simulink model "ESP_TCP_scoring"  (R2023a)
settings: Solver=FixedStepAuto  StartTime=0.0  StopTime=90  FixedStep=1  RelTol=1e-3
libraries: simulink x61, instrumentlib x2, dspsigattribs x1, dspstat3 x1, slrealtimeiplib x1
settings Model: SimulationMode=accelerator  PacingRate=6  Creator=Acer  LastModifiedBy=Acer

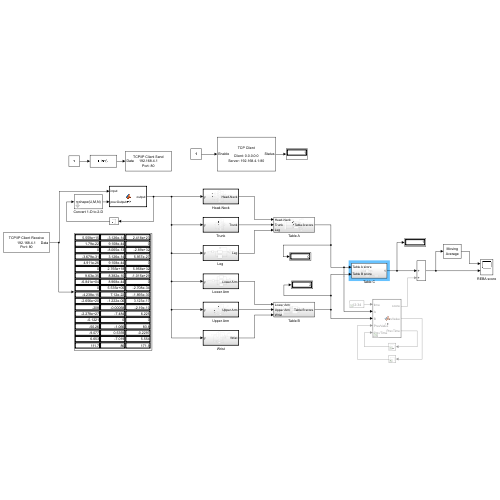
[thumbnail: Simulink's stored preview of the top-level diagram]
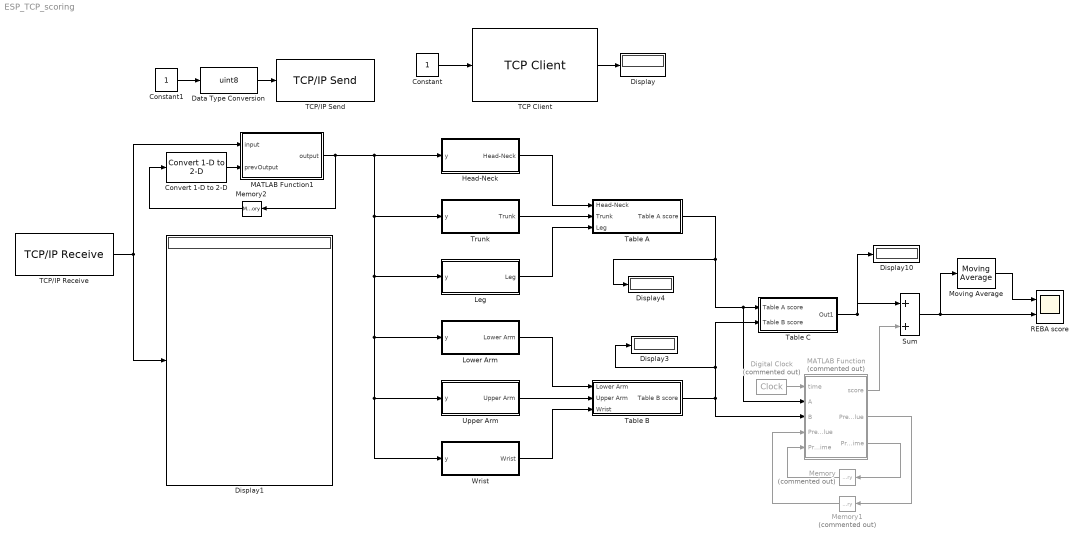
== system ESP_TCP_scoring ==
  Constant : Constant
  Constant1 : Constant
  Convert 1-D to 2-D : dspsigattribs/Convert 1-D to 2-D  M=1  N=54  frameBasedOut=off
      settings: LibrarySourceBlock=dsphdlsupportsigmgmt/Convert 1-D to 2-D
  Data Type Conversion : DataTypeConversion  OutDataTypeStr=uint8  SaturateOnIntegerOverflow=off  RndMeth=Floor
  Digital Clock : DigitalClock  Commented=on
  Display{,1,3..4,10} (5 alike) : Display
  Head-Neck : Subsystem  TreatAsAtomicUnit=on
  "Leg " : Subsystem  TreatAsAtomicUnit=on
  Lower Arm : Subsystem  TreatAsAtomicUnit=on
  MATLAB Function : MATLAB Function  Commented=on  TreatAsAtomicUnit=on
  MATLAB Function1 : MATLAB Function  TreatAsAtomicUnit=on
  Memory : Memory  Commented=on
  Memory1 : Memory  Commented=on
  Memory2 : Memory  InitialCondition=zeros(1,54)
  Moving Average : dspstat3/Moving Average  Method=Sliding window  ForgettingFactorPort=off  SpecifyWindowLength=on  WindowLength=4  OverlapLength=3  AllowArbitraryInputLength=off  ForgettingFactor=0.9  SimulateUsing=Code generation
  REBA score : Scope  NumInputPorts=2
  Sum : Sum  Inputs=|++
  TCP Client : slrealtimeiplib/TCP Client  Priority=-1  useHostTargetConn=off  remoteAddress=192.168.4.1  remotePort=80
  TCP/IP Receive : instrumentlib/TCP//IP Receive  Host=192.168.4.1  Port=80  DataSize=[ 1, 54]  DataType=double  ASCIIFormatting=%f  Terminator=LF  CustomTerminator=10  ByteOrder=little-endian  EnableBlockingMode=on  Timeout=20  SampleTime=1  SimulateUsing=Interpreted execution
  TCP/IP Send : instrumentlib/TCP//IP Send  Host=192.168.4.1  Port=80  ByteOrder=big-endian  EnableBlockingMode=on  Timeout=20  TransferDelay=on  SimulateUsing=Interpreted execution
  Table A : Subsystem
  Table B : Subsystem
  Table C : Subsystem
  Trunk : Subsystem  TreatAsAtomicUnit=on
  Upper Arm : Subsystem  TreatAsAtomicUnit=on
  Wrist : Subsystem  TreatAsAtomicUnit=on
  wires:
  Constant1/1 -> Data Type Conversion/1
  Constant/1 -> TCP Client/1
  Data Type Conversion/1 -> TCP/IP Send/1
  TCP Client/1 -> Display/1
  TCP/IP Receive/1 -> Display1/1, MATLAB Function1/1(input)
  Head-Neck/1(Head-Neck) -> Table A/1(Head-Neck)
  Trunk/1(Trunk) -> Table A/2(Trunk)
  "Leg "/1(Leg) -> Table A/3(Leg)
  Lower Arm/1(Lower Arm) -> Table B/1(Lower Arm)
  Upper Arm/1(Upper Arm) -> Table B/2(Upper Arm)
  Wrist/1(Wrist) -> Table B/3(Wrist)
  Table A/1(Table A score) -> Display4/1, MATLAB Function/2(A), Table C/1(Table A score)
  Table B/1(Table B score) -> MATLAB Function/3(B), Display3/1, Table C/2(Table B score)
  MATLAB Function/1(score) -> Sum/2
  Digital Clock/1 -> MATLAB Function/1(time)
  MATLAB Function/3(PrevTime) -> Memory/1
  Memory/1 -> MATLAB Function/5("PrevTime ")
  Memory1/1 -> MATLAB Function/4("PrevValue ")
  MATLAB Function/2(PrevValue) -> Memory1/1
  MATLAB Function1/1(output) -> Memory2/1, "Leg "/1(y), Lower Arm/1(y), Wrist/1(y), Upper Arm/1(y), Trunk/1(y), Head-Neck/1(y)
  Convert 1-D to 2-D/1 -> MATLAB Function1/2(prevOutput)
  Memory2/1 -> Convert 1-D to 2-D/1
  Table C/1(Out1) -> Sum/1, Display10/1
  Moving Average/1 -> REBA score/1
  Sum/1 -> Moving Average/1, REBA score/2

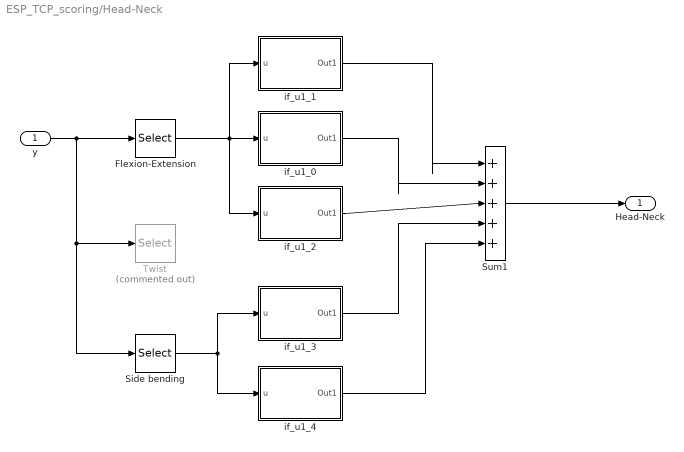
== system ESP_TCP_scoring/Head-Neck ==
  y : Inport
  Flexion-Extension : Selector  NumberOfDimensions=2  InputPortWidth=3  IndexOptions=Index vector (dialog),Index vector (dialog)  Indices=1,7  OutputSizes=1,1
  Side bending : Selector  NumberOfDimensions=2  InputPortWidth=3  IndexOptions=Index vector (dialog),Index vector (dialog)  Indices=1,1  OutputSizes=1,1
  Sum1 : Sum  Inputs=|+++++
  Twist : Selector  Commented=on  NumberOfDimensions=2  InputPortWidth=3  IndexOptions=Index vector (dialog),Index vector (dialog)  Indices=1,7  OutputSizes=1,1
  if_u1_0 : Subsystem  mask{a=69, b=1, c=2}
      mask prompts: a "u1 less then or equal to"; b "u1 greater then or equal to"; c "Constant"
      mask Display: text(5, 10, 'Gain');
  if_u1_1 : Subsystem  mask{a=80, b=70, c=1}
      mask prompts: a "u1 less then or equal to"; b "u1 greater then or equal to"; c "Constant"
      mask Display: text(5, 10, 'Gain');
  if_u1_2 : Subsystem  mask{a=180, b=100, c=2}
      mask prompts: a "u1 less then or equal to"; b "u1 greater then or equal to"; c "Constant"
      mask Display: text(5, 10, 'Gain');
  if_u1_3 : Subsystem  mask{a=-4.15, b=-9.81, c=1}
      mask prompts: a "u1 less then or equal to"; b "u1 greater then or equal to"; c "Constant"
      mask Display: text(5, 10, 'Gain');
  if_u1_4 : Subsystem  mask{a=9.81, b=4.15, c=1}
      mask prompts: a "u1 less then or equal to"; b "u1 greater then or equal to"; c "Constant"
      mask Display: text(5, 10, 'Gain');
  Head-Neck : Outport
  wires:
  y/1 -> Twist/1, Side bending/1, Flexion-Extension/1
  Flexion-Extension/1 -> if_u1_2/1(u), if_u1_0/1(u), if_u1_1/1(u)
  Side bending/1 -> if_u1_4/1(u), if_u1_3/1(u)
  if_u1_1/1(Out1) -> Sum1/1
  if_u1_0/1(Out1) -> Sum1/2
  if_u1_2/1(Out1) -> Sum1/3
  if_u1_3/1(Out1) -> Sum1/4
  if_u1_4/1(Out1) -> Sum1/5
  Sum1/1 -> Head-Neck/1

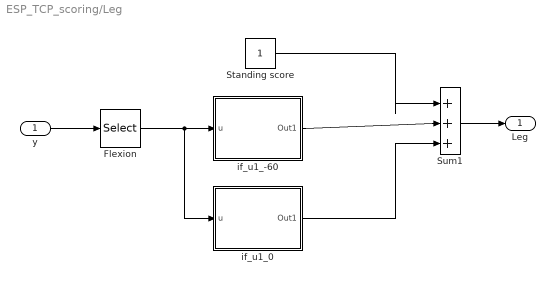
== system ESP_TCP_scoring/Leg  ==
  y : Inport
  Flexion : Selector  NumberOfDimensions=2  InputPortWidth=3  IndexOptions=Index vector (dialog),Index vector (dialog)  Indices=1,25  OutputSizes=1,1
  Standing score : Constant
  Sum1 : Sum  Inputs=|+++
  if_u1_-60 : Subsystem  mask{a=-60, b=-85, c=1}
      mask prompts: a "u1 less then or equal to"; b "u1 greater then or equal to"; c "Constant"
      mask Display: text(5, 10, 'Gain');
  if_u1_0 : Subsystem  mask{a=0, b=-59, c=2}
      mask prompts: a "u1 less then or equal to"; b "u1 greater then or equal to"; c "Constant"
      mask Display: text(5, 10, 'Gain');
  Leg : Outport
  wires:
  Standing score/1 -> Sum1/1
  y/1 -> Flexion/1
  Flexion/1 -> if_u1_0/1(u), if_u1_-60/1(u)
  if_u1_-60/1(Out1) -> Sum1/2
  if_u1_0/1(Out1) -> Sum1/3
  Sum1/1 -> Leg/1

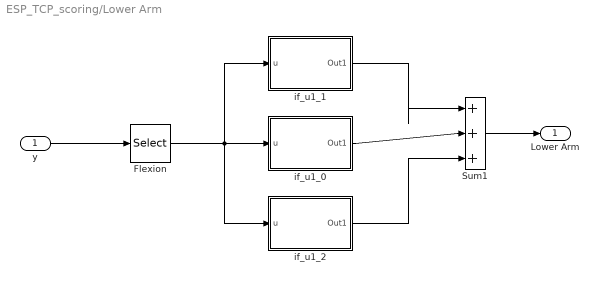
== system ESP_TCP_scoring/Lower Arm ==
  y : Inport
  Flexion : Selector  NumberOfDimensions=2  InputPortWidth=3  IndexOptions=Index vector (dialog),Index vector (dialog)  Indices=1,29  OutputSizes=1,1
  Sum1 : Sum  Inputs=|+++
  if_u1_0 : Subsystem  mask{a=9.81, b=1.71, c=2}
      mask prompts: a "u1 less then or equal to"; b "u1 greater then or equal to"; c "Constant"
      mask Display: text(5, 10, 'Gain');
  if_u1_1 : Subsystem  mask{a=1.70, b=-4.91, c=1}
      mask prompts: a "u1 less then or equal to"; b "u1 greater then or equal to"; c "Constant"
      mask Display: text(5, 10, 'Gain');
  if_u1_2 : Subsystem  mask{a=-4.91, b=-9.81, c=2}
      mask prompts: a "u1 less then or equal to"; b "u1 greater then or equal to"; c "Constant"
      mask Display: text(5, 10, 'Gain');
  Lower Arm : Outport
  wires:
  y/1 -> Flexion/1
  Flexion/1 -> if_u1_1/1(u), if_u1_0/1(u), if_u1_2/1(u)
  Sum1/1 -> Lower Arm/1
  if_u1_2/1(Out1) -> Sum1/3
  if_u1_0/1(Out1) -> Sum1/2
  if_u1_1/1(Out1) -> Sum1/1

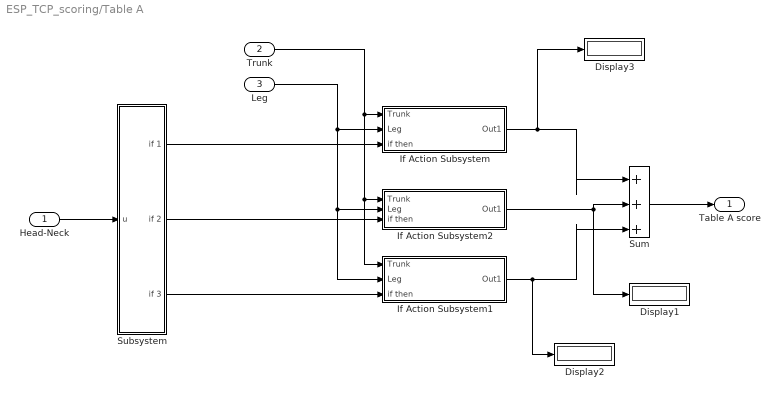
== system ESP_TCP_scoring/Table A ==
  Head-Neck : Inport
  Trunk : Inport  Port=2
  Leg : Inport  Port=3
  Display1 : Display
  Display2 : Display
  Display3 : Display
  If Action Subsystem : Subsystem  TreatAsAtomicUnit=on
  If Action Subsystem1 : Subsystem  TreatAsAtomicUnit=on
  If Action Subsystem2 : Subsystem  TreatAsAtomicUnit=on
  Subsystem : Subsystem
  Sum : Sum  Inputs=|+++
  Table A score : Outport
  wires:
  Trunk/1 -> If Action Subsystem1/1(Trunk), If Action Subsystem2/1(Trunk), If Action Subsystem/1(Trunk)
  Leg/1 -> If Action Subsystem1/2(Leg), If Action Subsystem2/2(Leg), If Action Subsystem/2(Leg)
  Sum/1 -> Table A score/1
  If Action Subsystem/1(Out1) -> Display3/1, Sum/1
  If Action Subsystem1/1(Out1) -> Display2/1, Sum/3
  Head-Neck/1 -> Subsystem/1(u)
  Subsystem/1(if 1) -> If Action Subsystem/3(if then)
  Subsystem/2(if 2) -> If Action Subsystem2/3(if then)
  Subsystem/3(if 3) -> If Action Subsystem1/3(if then)
  If Action Subsystem2/1(Out1) -> Display1/1, Sum/2

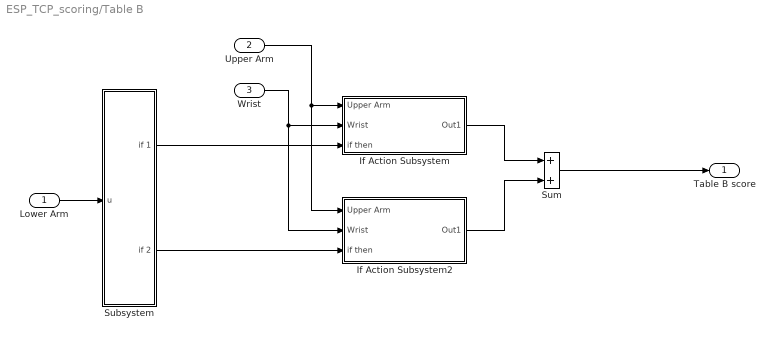
== system ESP_TCP_scoring/Table B ==
  Lower Arm : Inport
  Upper Arm : Inport  Port=2
  Wrist : Inport  Port=3
  If Action Subsystem : Subsystem  TreatAsAtomicUnit=on
  If Action Subsystem2 : Subsystem  TreatAsAtomicUnit=on
  Subsystem : Subsystem
  Sum : Sum
  Table B score : Outport
  wires:
  Upper Arm/1 -> If Action Subsystem2/1(Upper Arm), If Action Subsystem/1(Upper Arm)
  Wrist/1 -> If Action Subsystem2/2(Wrist), If Action Subsystem/2(Wrist)
  If Action Subsystem/1(Out1) -> Sum/1
  If Action Subsystem2/1(Out1) -> Sum/2
  Lower Arm/1 -> Subsystem/1(u)
  Subsystem/1(if 1) -> If Action Subsystem/3(if then)
  Subsystem/2(if 2) -> If Action Subsystem2/3(if then)
  Sum/1 -> Table B score/1

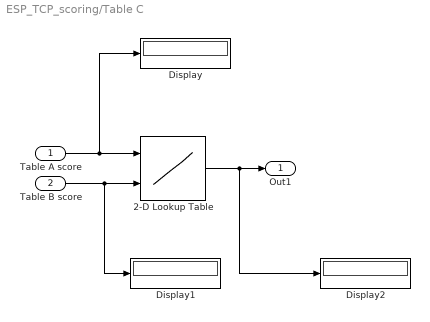
== system ESP_TCP_scoring/Table C ==
  Table A score : Inport
  Table B score : Inport  Port=2
  2-D Lookup Table : Lookup_n-D  BreakpointsForDimension1=[0:12]  BreakpointsForDimension2=[0:12]  Table=[1 1 1 1 1 1 1 1 1 1 1 1 1; 1 1 1 1 2 3 3 4 5 6 7 7 7; 1 1 2 2 3 4 4 5 6 6 7 7 8; 1 2 3 3 3 4 5 6 7 7 8 8 8; 1 3 4 4 4 5 6 7 8 8 9 9 9; 1 4 4 4 5 6 7 8 8 9 9 9 9; 1 6 6 6 7 8 8 9 9 10 10 10 10; 1 7 7 7 8 9 9 9 10 10 11 11 11; 1 8 8 8 9 10 10 10 10 10 11 11 11; 1 9 9 9 10 10 10 11 11 11 12 12 12; 1 10 10 10 11 11 11 11 12 12 12 12 12; 1 11 11 11 11 12 12 12 12 12 12 12 12; 1 12 12 12 12 12 12 12 12 12 12 12 12]  OutDataTypeStr=Inherit: Inherit from 'Table data'  RndMeth=Simplest
      settings: InputPortMap=u0,u1
  Display : Display
  Display1 : Display
  Display2 : Display
  Out1 : Outport
  wires:
  Table A score/1 -> Display/1, 2-D Lookup Table/1
  Table B score/1 -> Display1/1, 2-D Lookup Table/2
  2-D Lookup Table/1 -> Display2/1, Out1/1

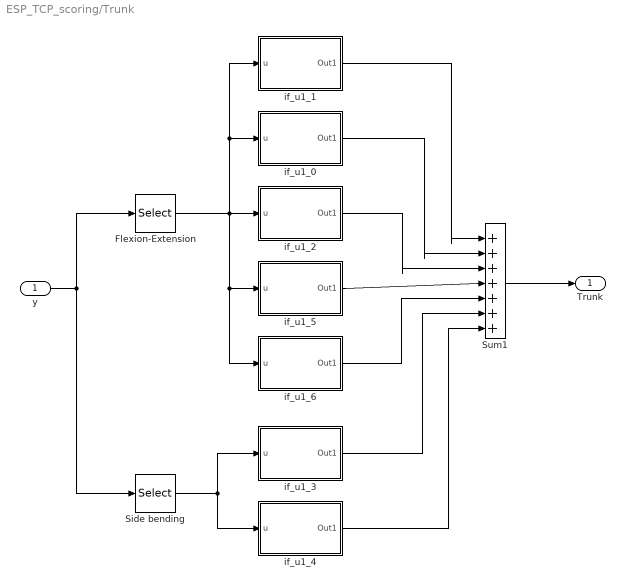
== system ESP_TCP_scoring/Trunk ==
  y : Inport
  Flexion-Extension : Selector  NumberOfDimensions=2  InputPortWidth=3  IndexOptions=Index vector (dialog),Index vector (dialog)  Indices=1,16  OutputSizes=1,1
  Side bending : Selector  NumberOfDimensions=2  InputPortWidth=3  IndexOptions=Index vector (dialog),Index vector (dialog)  Indices=1,17  OutputSizes=1,1
  Sum1 : Sum  Inputs=|+++++++
  if_u1_0 : Subsystem  mask{a=-96, b=-180, c=2}
      mask prompts: a "u1 less then or equal to"; b "u1 greater then or equal to"; c "Constant"
      mask Display: text(5, 10, 'Gain');
  if_u1_1 : Subsystem  mask{a=-85, b=-95, c=1}
      mask prompts: a "u1 less then or equal to"; b "u1 greater then or equal to"; c "Constant"
      mask Display: text(5, 10, 'Gain');
  if_u1_2 : Subsystem  mask{a=-70, b=-84, c=2}
      mask prompts: a "u1 less then or equal to"; b "u1 greater then or equal to"; c "Constant"
      mask Display: text(5, 10, 'Gain');
  if_u1_3 : Subsystem  mask{a=90, b=15, c=1}
      mask prompts: a "u1 less then or equal to"; b "u1 greater then or equal to"; c "Constant"
      mask Display: text(5, 10, 'Gain');
  if_u1_4 : Subsystem  mask{a=-15, b=-90, c=1}
      mask prompts: a "u1 less then or equal to"; b "u1 greater then or equal to"; c "Constant"
      mask Display: text(5, 10, 'Gain');
  if_u1_5 : Subsystem  mask{a=-30, b=-71, c=3}
      mask prompts: a "u1 less then or equal to"; b "u1 greater then or equal to"; c "Constant"
      mask Display: text(5, 10, 'Gain');
  if_u1_6 : Subsystem  mask{a=0, b=-29, c=4}
      mask prompts: a "u1 less then or equal to"; b "u1 greater then or equal to"; c "Constant"
      mask Display: text(5, 10, 'Gain');
  Trunk : Outport
  wires:
  y/1 -> Flexion-Extension/1, Side bending/1
  Flexion-Extension/1 -> if_u1_6/1(u), if_u1_5/1(u), if_u1_0/1(u), if_u1_1/1(u), if_u1_2/1(u)
  Sum1/1 -> Trunk/1
  Side bending/1 -> if_u1_4/1(u), if_u1_3/1(u)
  if_u1_1/1(Out1) -> Sum1/1
  if_u1_0/1(Out1) -> Sum1/2
  if_u1_2/1(Out1) -> Sum1/3
  if_u1_5/1(Out1) -> Sum1/4
  if_u1_6/1(Out1) -> Sum1/5
  if_u1_3/1(Out1) -> Sum1/6
  if_u1_4/1(Out1) -> Sum1/7

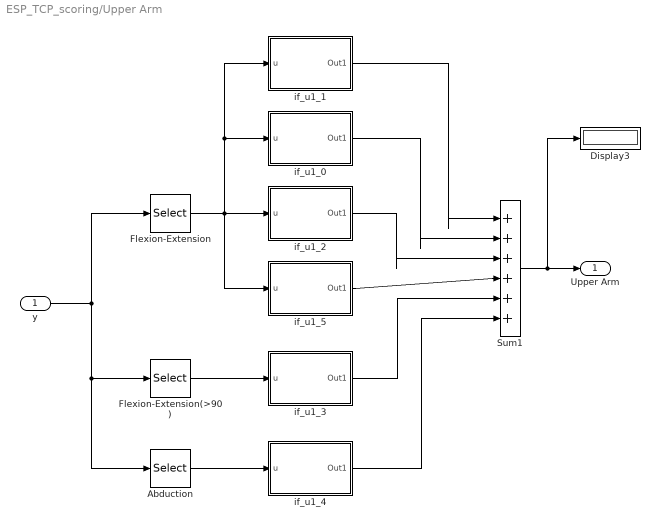
== system ESP_TCP_scoring/Upper Arm ==
  y : Inport
  Abduction : Selector  NumberOfDimensions=2  InputPortWidth=3  IndexOptions=Index vector (dialog),Index vector (dialog)  Indices=1,39  OutputSizes=1,1
  Display3 : Display
  Flexion-Extension : Selector  NumberOfDimensions=2  InputPortWidth=3  IndexOptions=Index vector (dialog),Index vector (dialog)  Indices=1,37  OutputSizes=1,1
  Flexion-Extension(>90) : Selector  NumberOfDimensions=2  InputPortWidth=3  IndexOptions=Index vector (dialog),Index vector (dialog)  Indices=1,38  OutputSizes=1,1
  Sum1 : Sum  Inputs=|++++++
  if_u1_0 : Subsystem  mask{a=9.81, b=3.36, c=2}
      mask prompts: a "u1 less then or equal to"; b "u1 greater then or equal to"; c "Constant"
      mask Display: text(5, 10, 'Gain');
  if_u1_1 : Subsystem  mask{a=3.35, b=-3.35, c=1}
      mask prompts: a "u1 less then or equal to"; b "u1 greater then or equal to"; c "Constant"
      mask Display: text(5, 10, 'Gain');
  if_u1_2 : Subsystem  mask{a=-3.36, b=-6.93, c=2}
      mask prompts: a "u1 less then or equal to"; b "u1 greater then or equal to"; c "Constant"
      mask Display: text(5, 10, 'Gain');
  if_u1_3 : Subsystem  mask{a=9, b=3, c=4}
      mask prompts: a "u1 less then or equal to"; b "u1 greater then or equal to"; c "Constant"
      mask Display: text(5, 10, 'Gain');
  if_u1_4 : Subsystem  mask{a=9.81, b=6.30, c=1}
      mask prompts: a "u1 less then or equal to"; b "u1 greater then or equal to"; c "Constant"
      mask Display: text(5, 10, 'Gain');
  if_u1_5 : Subsystem  mask{a=-6.94, b=-9.81, c=3}
      mask prompts: a "u1 less then or equal to"; b "u1 greater then or equal to"; c "Constant"
      mask Display: text(5, 10, 'Gain');
  Upper Arm : Outport
  wires:
  y/1 -> Flexion-Extension/1, Flexion-Extension(>90)/1, Abduction/1
  Flexion-Extension/1 -> if_u1_1/1(u), if_u1_0/1(u), if_u1_5/1(u), if_u1_2/1(u)
  Sum1/1 -> Display3/1, Upper Arm/1
  Abduction/1 -> if_u1_4/1(u)
  Flexion-Extension(>90)/1 -> if_u1_3/1(u)
  if_u1_1/1(Out1) -> Sum1/1
  if_u1_0/1(Out1) -> Sum1/2
  if_u1_2/1(Out1) -> Sum1/3
  if_u1_5/1(Out1) -> Sum1/4
  if_u1_3/1(Out1) -> Sum1/5
  if_u1_4/1(Out1) -> Sum1/6

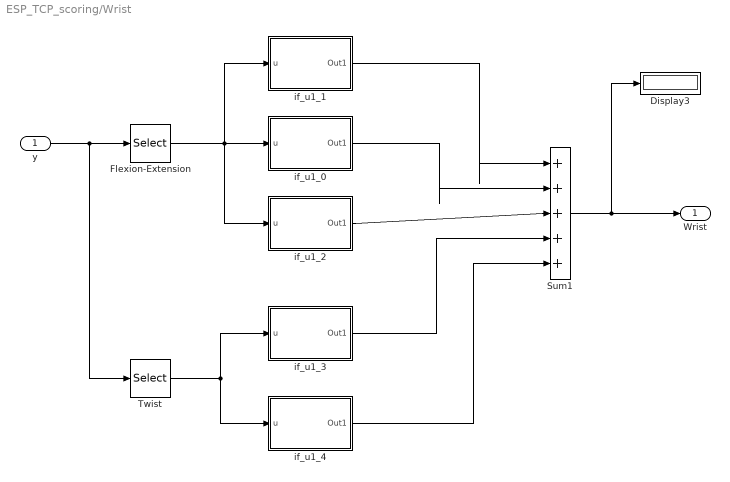
== system ESP_TCP_scoring/Wrist ==
  y : Inport
  Display3 : Display
  Flexion-Extension : Selector  NumberOfDimensions=2  InputPortWidth=3  IndexOptions=Index vector (dialog),Index vector (dialog)  Indices=1,47  OutputSizes=1,1
  Sum1 : Sum  Inputs=|+++++
  Twist : Selector  NumberOfDimensions=2  InputPortWidth=3  IndexOptions=Index vector (dialog),Index vector (dialog)  Indices=1,53  OutputSizes=1,1
  if_u1_0 : Subsystem  mask{a=9.81, b=2.54, c=2}
      mask prompts: a "u1 less then or equal to"; b "u1 greater then or equal to"; c "Constant"
      mask Display: text(5, 10, 'Gain');
  if_u1_1 : Subsystem  mask{a=2.53, b=-2.53, c=1}
      mask prompts: a "u1 less then or equal to"; b "u1 greater then or equal to"; c "Constant"
      mask Display: text(5, 10, 'Gain');
  if_u1_2 : Subsystem  mask{a=-2.54, b=-9.81, c=2}
      mask prompts: a "u1 less then or equal to"; b "u1 greater then or equal to"; c "Constant"
      mask Display: text(5, 10, 'Gain');
  if_u1_3 : Subsystem  mask{a=90, b=45, c=1}
      mask prompts: a "u1 less then or equal to"; b "u1 greater then or equal to"; c "Constant"
      mask Display: text(5, 10, 'Gain');
  if_u1_4 : Subsystem  mask{a=-45, b=-90, c=1}
      mask prompts: a "u1 less then or equal to"; b "u1 greater then or equal to"; c "Constant"
      mask Display: text(5, 10, 'Gain');
  Wrist : Outport
  wires:
  y/1 -> Flexion-Extension/1, Twist/1
  Flexion-Extension/1 -> if_u1_1/1(u), if_u1_0/1(u), if_u1_2/1(u)
  Sum1/1 -> Display3/1, Wrist/1
  if_u1_2/1(Out1) -> Sum1/3
  if_u1_0/1(Out1) -> Sum1/2
  if_u1_1/1(Out1) -> Sum1/1
  Twist/1 -> if_u1_3/1(u), if_u1_4/1(u)
  if_u1_3/1(Out1) -> Sum1/4
  if_u1_4/1(Out1) -> Sum1/5

== system ESP_TCP_scoring/Head-Neck/if_u1_0 ==
  u : Inport
  Compare To Constant : simulink/Logic and Bit Operations/Compare To Constant  relop=<=  const=a  OutDataTypeStr=boolean
  Compare To Constant1 : simulink/Logic and Bit Operations/Compare To Constant  relop=>=  const=b  OutDataTypeStr=boolean
  Constant2 : Constant  Value=c
  Product : Product
  Product1 : Product
  Out1 : Outport
  wires:
  Product1/1 -> Out1/1
  Compare To Constant1/1 -> Product/2
  Compare To Constant/1 -> Product/1
  Product/1 -> Product1/1
  Constant2/1 -> Product1/2
  u/1 -> Compare To Constant1/1, Compare To Constant/1

== system ESP_TCP_scoring/Head-Neck/if_u1_1 ==
  u : Inport
  Compare To Constant : simulink/Logic and Bit Operations/Compare To Constant  relop=<=  const=a  OutDataTypeStr=boolean
  Compare To Constant1 : simulink/Logic and Bit Operations/Compare To Constant  relop=>=  const=b  OutDataTypeStr=boolean
  Constant2 : Constant  Value=c
  Product : Product
  Product1 : Product
  Out1 : Outport
  wires:
  Product1/1 -> Out1/1
  Compare To Constant1/1 -> Product/2
  Compare To Constant/1 -> Product/1
  Product/1 -> Product1/1
  Constant2/1 -> Product1/2
  u/1 -> Compare To Constant1/1, Compare To Constant/1

== system ESP_TCP_scoring/Head-Neck/if_u1_2 ==
  u : Inport
  Compare To Constant : simulink/Logic and Bit Operations/Compare To Constant  relop=<=  const=a  OutDataTypeStr=boolean
  Compare To Constant1 : simulink/Logic and Bit Operations/Compare To Constant  relop=>=  const=b  OutDataTypeStr=boolean
  Constant2 : Constant  Value=c
  Product : Product
  Product1 : Product
  Out1 : Outport
  wires:
  Product1/1 -> Out1/1
  Compare To Constant1/1 -> Product/2
  Compare To Constant/1 -> Product/1
  Product/1 -> Product1/1
  Constant2/1 -> Product1/2
  u/1 -> Compare To Constant1/1, Compare To Constant/1

== system ESP_TCP_scoring/Head-Neck/if_u1_3 ==
  u : Inport
  Compare To Constant : simulink/Logic and Bit Operations/Compare To Constant  relop=<=  const=a  OutDataTypeStr=boolean
  Compare To Constant1 : simulink/Logic and Bit Operations/Compare To Constant  relop=>=  const=b  OutDataTypeStr=boolean
  Constant2 : Constant  Value=c
  Product : Product
  Product1 : Product
  Out1 : Outport
  wires:
  Product1/1 -> Out1/1
  Compare To Constant1/1 -> Product/2
  Compare To Constant/1 -> Product/1
  Product/1 -> Product1/1
  Constant2/1 -> Product1/2
  u/1 -> Compare To Constant1/1, Compare To Constant/1

== system ESP_TCP_scoring/Head-Neck/if_u1_4 ==
  u : Inport
  Compare To Constant : simulink/Logic and Bit Operations/Compare To Constant  relop=<=  const=a  OutDataTypeStr=boolean
  Compare To Constant1 : simulink/Logic and Bit Operations/Compare To Constant  relop=>=  const=b  OutDataTypeStr=boolean
  Constant2 : Constant  Value=c
  Product : Product
  Product1 : Product
  Out1 : Outport
  wires:
  Product1/1 -> Out1/1
  Compare To Constant1/1 -> Product/2
  Compare To Constant/1 -> Product/1
  Product/1 -> Product1/1
  Constant2/1 -> Product1/2
  u/1 -> Compare To Constant1/1, Compare To Constant/1

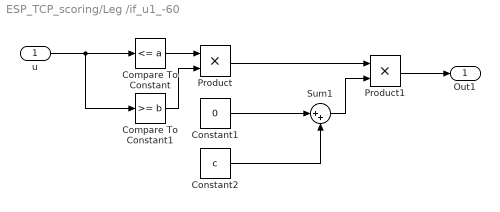
== system ESP_TCP_scoring/Leg /if_u1_-60 ==
  u : Inport
  Compare To Constant : simulink/Logic and Bit Operations/Compare To Constant  relop=<=  const=a  OutDataTypeStr=boolean
  Compare To Constant1 : simulink/Logic and Bit Operations/Compare To Constant  relop=>=  const=b  OutDataTypeStr=boolean
  Constant1 : Constant  Value=0
  Constant2 : Constant  Value=c
  Product : Product
  Product1 : Product
  Sum1 : Sum  Inputs=|++
  Out1 : Outport
  wires:
  Product1/1 -> Out1/1
  Compare To Constant1/1 -> Product/2
  Compare To Constant/1 -> Product/1
  Constant2/1 -> Sum1/2
  Constant1/1 -> Sum1/1
  Product/1 -> Product1/1
  Sum1/1 -> Product1/2
  u/1 -> Compare To Constant1/1, Compare To Constant/1

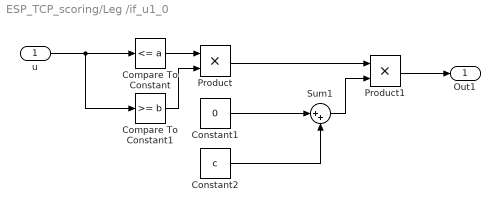
== system ESP_TCP_scoring/Leg /if_u1_0 ==
  u : Inport
  Compare To Constant : simulink/Logic and Bit Operations/Compare To Constant  relop=<=  const=a  OutDataTypeStr=boolean
  Compare To Constant1 : simulink/Logic and Bit Operations/Compare To Constant  relop=>=  const=b  OutDataTypeStr=boolean
  Constant1 : Constant  Value=0
  Constant2 : Constant  Value=c
  Product : Product
  Product1 : Product
  Sum1 : Sum  Inputs=|++
  Out1 : Outport
  wires:
  Product1/1 -> Out1/1
  Compare To Constant1/1 -> Product/2
  Compare To Constant/1 -> Product/1
  Constant2/1 -> Sum1/2
  Constant1/1 -> Sum1/1
  Product/1 -> Product1/1
  Sum1/1 -> Product1/2
  u/1 -> Compare To Constant1/1, Compare To Constant/1

== system ESP_TCP_scoring/Lower Arm/if_u1_0 ==
  u : Inport
  Compare To Constant : simulink/Logic and Bit Operations/Compare To Constant  relop=<=  const=a  OutDataTypeStr=boolean
  Compare To Constant1 : simulink/Logic and Bit Operations/Compare To Constant  relop=>=  const=b  OutDataTypeStr=boolean
  Constant2 : Constant  Value=c
  Product : Product
  Product1 : Product
  Out1 : Outport
  wires:
  Product1/1 -> Out1/1
  Compare To Constant1/1 -> Product/2
  Compare To Constant/1 -> Product/1
  Product/1 -> Product1/1
  Constant2/1 -> Product1/2
  u/1 -> Compare To Constant1/1, Compare To Constant/1

== system ESP_TCP_scoring/Lower Arm/if_u1_1 ==
  u : Inport
  Compare To Constant : simulink/Logic and Bit Operations/Compare To Constant  relop=<=  const=a  OutDataTypeStr=boolean
  Compare To Constant1 : simulink/Logic and Bit Operations/Compare To Constant  relop=>=  const=b  OutDataTypeStr=boolean
  Constant2 : Constant  Value=c
  Product : Product
  Product1 : Product
  Out1 : Outport
  wires:
  Product1/1 -> Out1/1
  Compare To Constant1/1 -> Product/2
  Compare To Constant/1 -> Product/1
  Product/1 -> Product1/1
  Constant2/1 -> Product1/2
  u/1 -> Compare To Constant1/1, Compare To Constant/1

== system ESP_TCP_scoring/Lower Arm/if_u1_2 ==
  u : Inport
  Compare To Constant : simulink/Logic and Bit Operations/Compare To Constant  relop=<=  const=a  OutDataTypeStr=boolean
  Compare To Constant1 : simulink/Logic and Bit Operations/Compare To Constant  relop=>=  const=b  OutDataTypeStr=boolean
  Constant2 : Constant  Value=c
  Product : Product
  Product1 : Product
  Out1 : Outport
  wires:
  Product1/1 -> Out1/1
  Compare To Constant1/1 -> Product/2
  Compare To Constant/1 -> Product/1
  Product/1 -> Product1/1
  Constant2/1 -> Product1/2
  u/1 -> Compare To Constant1/1, Compare To Constant/1

== system ESP_TCP_scoring/Table A/If Action Subsystem ==
  Trunk : Inport
  Leg : Inport  Port=2
  if then : Inport  Port=3
  2-D Lookup Table : Lookup_n-D  BreakpointsForDimension1=[1 2 3 4 5]  BreakpointsForDimension2=[1 2 3 4]  Table=[1 2 3 4; 2 3 4 5; 2 4 5 6; 3 5 6 7; 4 6 7 8]  InternalRulePriority=Speed  RndMeth=Simplest
      settings: InputPortMap=u0,u1
  Product : Product
  Out1 : Outport
  wires:
  Trunk/1 -> 2-D Lookup Table/1
  Leg/1 -> 2-D Lookup Table/2
  2-D Lookup Table/1 -> Product/1
  Product/1 -> Out1/1
  if then/1 -> Product/2

== system ESP_TCP_scoring/Table A/If Action Subsystem1 ==
  Trunk : Inport
  Leg : Inport  Port=2
  if then : Inport  Port=3
  2-D Lookup Table : Lookup_n-D  BreakpointsForDimension1=[1 2 3 4 5]  BreakpointsForDimension2=[1 2 3 4]  Table=[3 3 5 6; 4 5 6 7; 5 6 7 8; 6 7 8 9; 7 8 9 9]  InternalRulePriority=Speed  RndMeth=Simplest
      settings: InputPortMap=u0,u1
  Product : Product
  Out1 : Outport
  wires:
  Leg/1 -> 2-D Lookup Table/2
  Trunk/1 -> 2-D Lookup Table/1
  2-D Lookup Table/1 -> Product/1
  Product/1 -> Out1/1
  if then/1 -> Product/2

== system ESP_TCP_scoring/Table A/If Action Subsystem2 ==
  Trunk : Inport
  Leg : Inport  Port=2
  if then : Inport  Port=3
  2-D Lookup Table : Lookup_n-D  BreakpointsForDimension1=[1 2 3 4 5]  BreakpointsForDimension2=[1 2 3 4]  Table=[1 2 3 4; 3 4 5 6; 4 5 6 7; 5 6 7 8; 6 7 8 9]  InternalRulePriority=Speed  OutMin=[0]  RndMeth=Simplest
      settings: InputPortMap=u0,u1
  Product : Product
  Out1 : Outport
  wires:
  Trunk/1 -> 2-D Lookup Table/1
  Leg/1 -> 2-D Lookup Table/2
  2-D Lookup Table/1 -> Product/1
  Product/1 -> Out1/1
  if then/1 -> Product/2

== system ESP_TCP_scoring/Table A/Subsystem ==
  u : Inport
  Compare To Constant : simulink/Logic and Bit Operations/Compare To Constant  relop===  const=1  OutDataTypeStr=boolean
  Compare To Constant1 : simulink/Logic and Bit Operations/Compare To Constant  relop===  const=2  OutDataTypeStr=boolean
  Compare To Constant2 : simulink/Logic and Bit Operations/Compare To Constant  relop===  const=3  OutDataTypeStr=boolean
  if 1 : Outport
  if 2 : Outport  Port=2
  if 3 : Outport  Port=3
  wires:
  u/1 -> Compare To Constant/1, Compare To Constant2/1, Compare To Constant1/1
  Compare To Constant/1 -> if 1/1
  Compare To Constant1/1 -> if 2/1
  Compare To Constant2/1 -> if 3/1

== system ESP_TCP_scoring/Table B/If Action Subsystem ==
  Upper Arm : Inport
  Wrist : Inport  Port=2
  if then : Inport  Port=3
  2-D Lookup Table : Lookup_n-D  BreakpointsForDimension1=[1 2 3 4 5 6]  BreakpointsForDimension2=[1 2 3]  Table=[1 2 2; 1 2 3; 3 4 5; 4 5 5; 6 7 8; 7 8 8]  InternalRulePriority=Speed  RndMeth=Simplest
      settings: InputPortMap=u0,u1
  Product : Product
  Out1 : Outport
  wires:
  Upper Arm/1 -> 2-D Lookup Table/1
  Wrist/1 -> 2-D Lookup Table/2
  2-D Lookup Table/1 -> Product/1
  if then/1 -> Product/2
  Product/1 -> Out1/1

== system ESP_TCP_scoring/Table B/If Action Subsystem2 ==
  Upper Arm : Inport
  Wrist : Inport  Port=2
  if then : Inport  Port=3
  2-D Lookup Table : Lookup_n-D  BreakpointsForDimension1=[1 2 3 4 5 6]  BreakpointsForDimension2=[1 2 3]  Table=[1 2 3; 2 3 4; 4 5 5; 5 6 7; 7 8 8; 8 9 9]  InternalRulePriority=Speed  RndMeth=Simplest
      settings: InputPortMap=u0,u1
  Product : Product
  Out1 : Outport
  wires:
  Upper Arm/1 -> 2-D Lookup Table/1
  Wrist/1 -> 2-D Lookup Table/2
  Product/1 -> Out1/1
  2-D Lookup Table/1 -> Product/1
  if then/1 -> Product/2

== system ESP_TCP_scoring/Table B/Subsystem ==
  u : Inport
  Compare To Constant : simulink/Logic and Bit Operations/Compare To Constant  relop===  const=1  OutDataTypeStr=boolean
  Compare To Constant1 : simulink/Logic and Bit Operations/Compare To Constant  relop===  const=2  OutDataTypeStr=boolean
  if 1 : Outport
  if 2 : Outport  Port=2
  wires:
  u/1 -> Compare To Constant1/1, Compare To Constant/1
  Compare To Constant/1 -> if 1/1
  Compare To Constant1/1 -> if 2/1

== system ESP_TCP_scoring/Trunk/if_u1_0 ==
  u : Inport
  Compare To Constant : simulink/Logic and Bit Operations/Compare To Constant  relop=<=  const=a  OutDataTypeStr=boolean
  Compare To Constant1 : simulink/Logic and Bit Operations/Compare To Constant  relop=>=  const=b  OutDataTypeStr=boolean
  Constant2 : Constant  Value=c
  Product : Product
  Product1 : Product
  Out1 : Outport
  wires:
  Product1/1 -> Out1/1
  Compare To Constant1/1 -> Product/2
  Compare To Constant/1 -> Product/1
  Product/1 -> Product1/1
  Constant2/1 -> Product1/2
  u/1 -> Compare To Constant1/1, Compare To Constant/1

== system ESP_TCP_scoring/Trunk/if_u1_1 ==
  u : Inport
  Compare To Constant : simulink/Logic and Bit Operations/Compare To Constant  relop=<=  const=a  OutDataTypeStr=boolean
  Compare To Constant1 : simulink/Logic and Bit Operations/Compare To Constant  relop=>=  const=b  OutDataTypeStr=boolean
  Constant2 : Constant  Value=c
  Product : Product
  Product1 : Product
  Out1 : Outport
  wires:
  Product1/1 -> Out1/1
  Compare To Constant1/1 -> Product/2
  Compare To Constant/1 -> Product/1
  Product/1 -> Product1/1
  Constant2/1 -> Product1/2
  u/1 -> Compare To Constant1/1, Compare To Constant/1

== system ESP_TCP_scoring/Trunk/if_u1_2 ==
  u : Inport
  Compare To Constant : simulink/Logic and Bit Operations/Compare To Constant  relop=<=  const=a  OutDataTypeStr=boolean
  Compare To Constant1 : simulink/Logic and Bit Operations/Compare To Constant  relop=>=  const=b  OutDataTypeStr=boolean
  Constant2 : Constant  Value=c
  Product : Product
  Product1 : Product
  Out1 : Outport
  wires:
  Product1/1 -> Out1/1
  Compare To Constant1/1 -> Product/2
  Compare To Constant/1 -> Product/1
  Product/1 -> Product1/1
  Constant2/1 -> Product1/2
  u/1 -> Compare To Constant1/1, Compare To Constant/1

== system ESP_TCP_scoring/Trunk/if_u1_3 ==
  u : Inport
  Compare To Constant : simulink/Logic and Bit Operations/Compare To Constant  relop=<=  const=a  OutDataTypeStr=boolean
  Compare To Constant1 : simulink/Logic and Bit Operations/Compare To Constant  relop=>=  const=b  OutDataTypeStr=boolean
  Constant2 : Constant  Value=c
  Product : Product
  Product1 : Product
  Out1 : Outport
  wires:
  Product1/1 -> Out1/1
  Compare To Constant1/1 -> Product/2
  Compare To Constant/1 -> Product/1
  Product/1 -> Product1/1
  Constant2/1 -> Product1/2
  u/1 -> Compare To Constant1/1, Compare To Constant/1

== system ESP_TCP_scoring/Trunk/if_u1_4 ==
  u : Inport
  Compare To Constant : simulink/Logic and Bit Operations/Compare To Constant  relop=<=  const=a  OutDataTypeStr=boolean
  Compare To Constant1 : simulink/Logic and Bit Operations/Compare To Constant  relop=>=  const=b  OutDataTypeStr=boolean
  Constant2 : Constant  Value=c
  Product : Product
  Product1 : Product
  Out1 : Outport
  wires:
  Product1/1 -> Out1/1
  Compare To Constant1/1 -> Product/2
  Compare To Constant/1 -> Product/1
  Product/1 -> Product1/1
  Constant2/1 -> Product1/2
  u/1 -> Compare To Constant1/1, Compare To Constant/1

== system ESP_TCP_scoring/Trunk/if_u1_5 ==
  u : Inport
  Compare To Constant : simulink/Logic and Bit Operations/Compare To Constant  relop=<=  const=a  OutDataTypeStr=boolean
  Compare To Constant1 : simulink/Logic and Bit Operations/Compare To Constant  relop=>=  const=b  OutDataTypeStr=boolean
  Constant2 : Constant  Value=c
  Product : Product
  Product1 : Product
  Out1 : Outport
  wires:
  Product1/1 -> Out1/1
  Compare To Constant1/1 -> Product/2
  Compare To Constant/1 -> Product/1
  Product/1 -> Product1/1
  Constant2/1 -> Product1/2
  u/1 -> Compare To Constant1/1, Compare To Constant/1

== system ESP_TCP_scoring/Trunk/if_u1_6 ==
  u : Inport
  Compare To Constant : simulink/Logic and Bit Operations/Compare To Constant  relop=<=  const=a  OutDataTypeStr=boolean
  Compare To Constant1 : simulink/Logic and Bit Operations/Compare To Constant  relop=>=  const=b  OutDataTypeStr=boolean
  Constant2 : Constant  Value=c
  Product : Product
  Product1 : Product
  Out1 : Outport
  wires:
  Product1/1 -> Out1/1
  Compare To Constant1/1 -> Product/2
  Compare To Constant/1 -> Product/1
  Product/1 -> Product1/1
  Constant2/1 -> Product1/2
  u/1 -> Compare To Constant1/1, Compare To Constant/1

== system ESP_TCP_scoring/Upper Arm/if_u1_0 ==
  u : Inport
  Compare To Constant : simulink/Logic and Bit Operations/Compare To Constant  relop=<=  const=a  OutDataTypeStr=boolean
  Compare To Constant1 : simulink/Logic and Bit Operations/Compare To Constant  relop=>=  const=b  OutDataTypeStr=boolean
  Constant2 : Constant  Value=c
  Product : Product
  Product1 : Product
  Out1 : Outport
  wires:
  Product1/1 -> Out1/1
  Compare To Constant1/1 -> Product/2
  Compare To Constant/1 -> Product/1
  Product/1 -> Product1/1
  Constant2/1 -> Product1/2
  u/1 -> Compare To Constant1/1, Compare To Constant/1

== system ESP_TCP_scoring/Upper Arm/if_u1_1 ==
  u : Inport
  Compare To Constant : simulink/Logic and Bit Operations/Compare To Constant  relop=<=  const=a  OutDataTypeStr=boolean
  Compare To Constant1 : simulink/Logic and Bit Operations/Compare To Constant  relop=>=  const=b  OutDataTypeStr=boolean
  Constant2 : Constant  Value=c
  Product : Product
  Product1 : Product
  Out1 : Outport
  wires:
  Product1/1 -> Out1/1
  Compare To Constant1/1 -> Product/2
  Compare To Constant/1 -> Product/1
  Product/1 -> Product1/1
  Constant2/1 -> Product1/2
  u/1 -> Compare To Constant1/1, Compare To Constant/1

== system ESP_TCP_scoring/Upper Arm/if_u1_2 ==
  u : Inport
  Compare To Constant : simulink/Logic and Bit Operations/Compare To Constant  relop=<=  const=a  OutDataTypeStr=boolean
  Compare To Constant1 : simulink/Logic and Bit Operations/Compare To Constant  relop=>=  const=b  OutDataTypeStr=boolean
  Constant2 : Constant  Value=c
  Product : Product
  Product1 : Product
  Out1 : Outport
  wires:
  Product1/1 -> Out1/1
  Compare To Constant1/1 -> Product/2
  Compare To Constant/1 -> Product/1
  Product/1 -> Product1/1
  Constant2/1 -> Product1/2
  u/1 -> Compare To Constant1/1, Compare To Constant/1

== system ESP_TCP_scoring/Upper Arm/if_u1_3 ==
  u : Inport
  Compare To Constant : simulink/Logic and Bit Operations/Compare To Constant  relop=<=  const=a  OutDataTypeStr=boolean
  Compare To Constant1 : simulink/Logic and Bit Operations/Compare To Constant  relop=>=  const=b  OutDataTypeStr=boolean
  Constant2 : Constant  Value=c
  Product : Product
  Product1 : Product
  Out1 : Outport
  wires:
  Product1/1 -> Out1/1
  Compare To Constant1/1 -> Product/2
  Compare To Constant/1 -> Product/1
  Product/1 -> Product1/1
  Constant2/1 -> Product1/2
  u/1 -> Compare To Constant1/1, Compare To Constant/1

== system ESP_TCP_scoring/Upper Arm/if_u1_4 ==
  u : Inport
  Compare To Constant : simulink/Logic and Bit Operations/Compare To Constant  relop=<=  const=a  OutDataTypeStr=boolean
  Compare To Constant1 : simulink/Logic and Bit Operations/Compare To Constant  relop=>=  const=b  OutDataTypeStr=boolean
  Constant2 : Constant  Value=c
  Product : Product
  Product1 : Product
  Out1 : Outport
  wires:
  Product1/1 -> Out1/1
  Compare To Constant1/1 -> Product/2
  Compare To Constant/1 -> Product/1
  Product/1 -> Product1/1
  Constant2/1 -> Product1/2
  u/1 -> Compare To Constant1/1, Compare To Constant/1

== system ESP_TCP_scoring/Upper Arm/if_u1_5 ==
  u : Inport
  Compare To Constant : simulink/Logic and Bit Operations/Compare To Constant  relop=<=  const=a  OutDataTypeStr=boolean
  Compare To Constant1 : simulink/Logic and Bit Operations/Compare To Constant  relop=>=  const=b  OutDataTypeStr=boolean
  Constant2 : Constant  Value=c
  Product : Product
  Product1 : Product
  Out1 : Outport
  wires:
  Product1/1 -> Out1/1
  Compare To Constant1/1 -> Product/2
  Compare To Constant/1 -> Product/1
  Product/1 -> Product1/1
  Constant2/1 -> Product1/2
  u/1 -> Compare To Constant1/1, Compare To Constant/1

== system ESP_TCP_scoring/Wrist/if_u1_0 ==
  u : Inport
  Compare To Constant : simulink/Logic and Bit Operations/Compare To Constant  relop=<=  const=a  OutDataTypeStr=boolean
  Compare To Constant1 : simulink/Logic and Bit Operations/Compare To Constant  relop=>=  const=b  OutDataTypeStr=boolean
  Constant2 : Constant  Value=c
  Product : Product
  Product1 : Product
  Out1 : Outport
  wires:
  Product1/1 -> Out1/1
  Compare To Constant1/1 -> Product/2
  Compare To Constant/1 -> Product/1
  Product/1 -> Product1/1
  Constant2/1 -> Product1/2
  u/1 -> Compare To Constant1/1, Compare To Constant/1

== system ESP_TCP_scoring/Wrist/if_u1_1 ==
  u : Inport
  Compare To Constant : simulink/Logic and Bit Operations/Compare To Constant  relop=<=  const=a  OutDataTypeStr=boolean
  Compare To Constant1 : simulink/Logic and Bit Operations/Compare To Constant  relop=>=  const=b  OutDataTypeStr=boolean
  Constant2 : Constant  Value=c
  Product : Product
  Product1 : Product
  Out1 : Outport
  wires:
  Product1/1 -> Out1/1
  Compare To Constant1/1 -> Product/2
  Compare To Constant/1 -> Product/1
  Product/1 -> Product1/1
  Constant2/1 -> Product1/2
  u/1 -> Compare To Constant1/1, Compare To Constant/1

== system ESP_TCP_scoring/Wrist/if_u1_2 ==
  u : Inport
  Compare To Constant : simulink/Logic and Bit Operations/Compare To Constant  relop=<=  const=a  OutDataTypeStr=boolean
  Compare To Constant1 : simulink/Logic and Bit Operations/Compare To Constant  relop=>=  const=b  OutDataTypeStr=boolean
  Constant2 : Constant  Value=c
  Product : Product
  Product1 : Product
  Out1 : Outport
  wires:
  Product1/1 -> Out1/1
  Compare To Constant1/1 -> Product/2
  Compare To Constant/1 -> Product/1
  Product/1 -> Product1/1
  Constant2/1 -> Product1/2
  u/1 -> Compare To Constant1/1, Compare To Constant/1

== system ESP_TCP_scoring/Wrist/if_u1_3 ==
  u : Inport
  Compare To Constant : simulink/Logic and Bit Operations/Compare To Constant  relop=<=  const=a  OutDataTypeStr=boolean
  Compare To Constant1 : simulink/Logic and Bit Operations/Compare To Constant  relop=>=  const=b  OutDataTypeStr=boolean
  Constant2 : Constant  Value=c
  Product : Product
  Product1 : Product
  Out1 : Outport
  wires:
  Product1/1 -> Out1/1
  Compare To Constant1/1 -> Product/2
  Compare To Constant/1 -> Product/1
  Product/1 -> Product1/1
  Constant2/1 -> Product1/2
  u/1 -> Compare To Constant1/1, Compare To Constant/1

== system ESP_TCP_scoring/Wrist/if_u1_4 ==
  u : Inport
  Compare To Constant : simulink/Logic and Bit Operations/Compare To Constant  relop=<=  const=a  OutDataTypeStr=boolean
  Compare To Constant1 : simulink/Logic and Bit Operations/Compare To Constant  relop=>=  const=b  OutDataTypeStr=boolean
  Constant2 : Constant  Value=c
  Product : Product
  Product1 : Product
  Out1 : Outport
  wires:
  Product1/1 -> Out1/1
  Compare To Constant1/1 -> Product/2
  Compare To Constant/1 -> Product/1
  Product/1 -> Product1/1
  Constant2/1 -> Product1/2
  u/1 -> Compare To Constant1/1, Compare To Constant/1

== matlab function ESP_TCP_scoring/MATLAB Function1 ==
  data: input input; output output; prevOutput input
function output = limit(input,prevOutput)
%output=input;
if (any(input>500) || any(input<-500))
    output=prevOutput;
    output = reshape(output,1,54);
else
    output = input;
    output = reshape(output,1,54);
end

== matlab function ESP_TCP_scoring/MATLAB Function ==
  data: time input; score output; A input; B input; PrevValue input; PrevTime input; PrevValue output; PrevTime output
function [score,PrevValue,PrevTime] = fcn(time, A, B, PrevValue,PrevTime)
NewValue =A+B;
if(PrevValue ~=NewValue)
    PrevValue=NewValue;
    PrevTime=time;
end
if((time-PrevTime) <=60)
    score =0;
else
    score = 1;
end
